simulink model "FDM"  (R2021a)
settings: Solver=VariableStepAuto  StartTime=0.0  StopTime=10.0  RelTol=1e-3
settings Model: Creator=Bharat Gunhalkar  LastModifiedBy=Bharat Gunhalkar

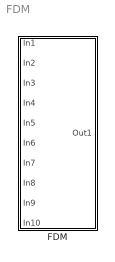
== system FDM ==
  FDM : Subsystem

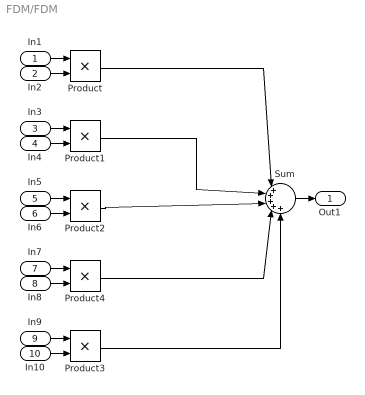
== system FDM/FDM ==
  In1 : Inport
  In2 : Inport  Port=2
  In3 : Inport  Port=3
  In4 : Inport  Port=4
  In5 : Inport  Port=5
  In6 : Inport  Port=6
  In7 : Inport  Port=7
  In8 : Inport  Port=8
  In9 : Inport  Port=9
  In10 : Inport  Port=10
  Product{,1..4} (5 alike) : Product
  Sum : Sum  Inputs=|+++++
  Out1 : Outport
  wires:
  Product1/1 -> Sum/2
  Product3/1 -> Sum/5
  Product4/1 -> Sum/4
  In2/1 -> Product/2
  Product/1 -> Sum/1
  Product2/1 -> Sum/3
  In1/1 -> Product/1
  In4/1 -> Product1/2
  In7/1 -> Product4/1
  In9/1 -> Product3/1
  In3/1 -> Product1/1
  In10/1 -> Product3/2
  In5/1 -> Product2/1
  Sum/1 -> Out1/1
  In6/1 -> Product2/2
  In8/1 -> Product4/2
